simulink model "gm_parallel_min_cost_function_vopt_6phase"  (R2022a)
settings: Solver=FixedStepDiscrete  StartTime=0.0  StopTime=10.0  RelTol=1e-3
undefined symbols (not defined in the file or in its folder): f_c
libraries: hdlmdlgenlib x368
(part 1 of 3)
settings Model: Creator=Andre Merx  LastModifiedBy=Andre Merx
settings SolverCC: AlgebraicLoopSolver=TrustRegion
settings DataIOCC: LimitDataPoints=on  SaveOutput=off  SaveTime=off
settings OptimizationCC: BlockReduction=off  ConditionallyExecuteInputs=off  DefaultParameterBehavior=Inlined  LifeSpan=inf
settings DebuggingCC: AlgebraicLoopMsg=error  InheritedTsInSrcMsg=none  SingleTaskRateTransMsg=error  UnconnectedInputMsg=warning  UnconnectedOutputMsg=warning  UnconnectedLineMsg=warning  AllowSymbolicDim=off  StrictBusMsg=ErrorOnBusTreatedAsVector  SFUnexpectedBacktrackingDiag=warning  SFNoUnconditionalDefaultTransitionDiag=warning  SFExecutionAtInitializationDiag=none  SFMachineParentedDataDiag=warning  ArithmeticOperatorsInVariantConditions=warning
settings HardwareCC: ProdBitPerPointer=32  ProdBitPerSizeT=32  ProdBitPerPtrDiffT=32  ProdLargestAtomicFloat=None  ProdIntDivRoundTo=Undefined  ProdEndianess=Unspecified  ProdWordSize=32  ProdHWDeviceType=ASIC/FPGA->ASIC/FPGA  ProdEqTarget=off
settings SFSimCC: SimUseLocalCustomCode=off  CustomCodeUndefinedFunction=UseInterfaceOnly
settings RTWCC: RTWUseLocalCustomCode=off
settings CodeAppCC: StateflowObjectComments=on
settings GRTTargetCC: TargetLangStandard=C89/C90 (ANSI)
settings ConfigComp: CovScope=ReferencedModels  CovMetricSettings=dw  CovSaveCumulativeToWorkspaceVar=on  CovSaveSingleToWorkspaceVar=on  CovExternalEMLEnable=off  CovSFcnEnable=off

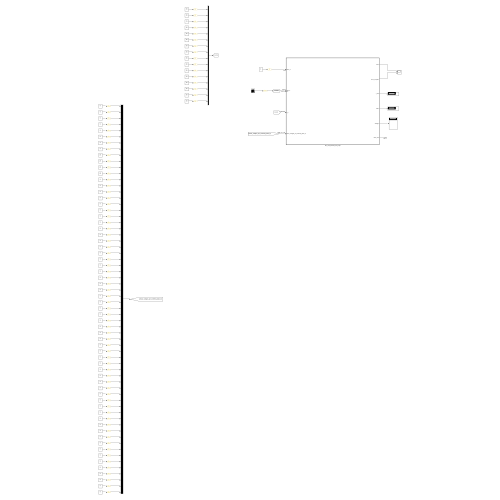
[thumbnail: Simulink's stored preview of the top-level diagram]
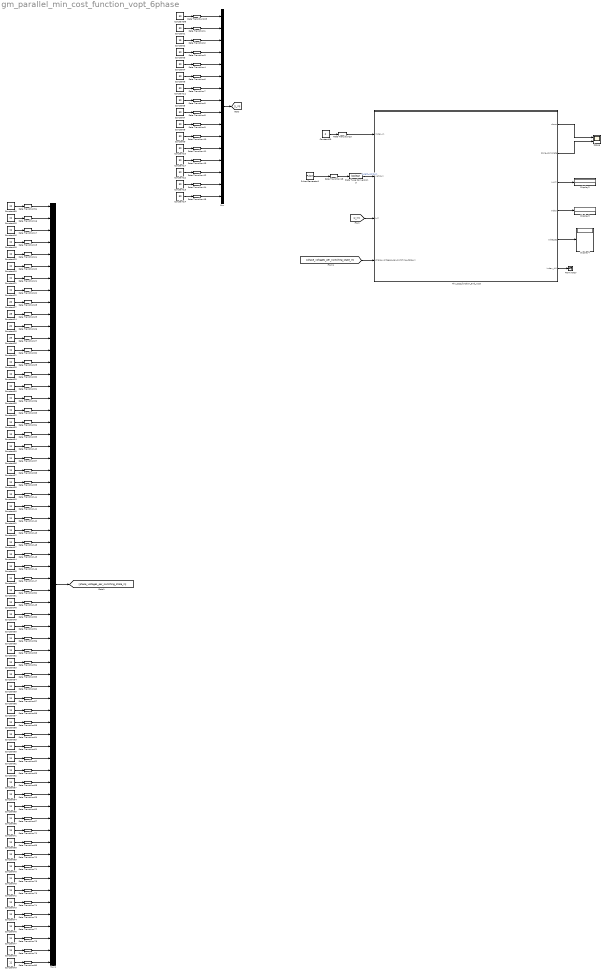
== system gm_parallel_min_cost_function_vopt_6phase ==
  Constant{1,3..14,17,98} (15 alike) : Constant  Value=30  OutDataTypeStr=fixdt(1,20,11)  SampleTime=-1
  Constant{15..16,18,20..23,28..79,89} (60 alike) : Constant  Value=11  OutDataTypeStr=fixdt(1,24,11)  SampleTime=-1  LockScale=on
  Constant19 : Constant  Value=4  OutDataTypeStr=int32  SampleTime=-1
  Constant2 : Constant  Value=15  OutDataTypeStr=fixdt(1,20,11)  SampleTime=-1
  Constant24 : Constant  Value=23  OutDataTypeStr=fixdt(1,24,11)  SampleTime=-1  LockScale=on
  Constant25 : Constant  Value=24  OutDataTypeStr=fixdt(1,24,11)  SampleTime=-1  LockScale=on
  Constant26 : Constant  Value=25  OutDataTypeStr=fixdt(1,24,11)  SampleTime=-1  LockScale=on
  Constant27 : Constant  Value=22  OutDataTypeStr=fixdt(1,24,11)  SampleTime=-1  LockScale=on
  Data Type Conversion3 : DataTypeConversion  OutDataTypeStr=boolean  SaturateOnIntegerOverflow=off  RndMeth=Floor
  Display2 : Display
  Display3 : Display
  Display4 : Display
  Min_cost_function_and_vopt : Subsystem  TreatAsAtomicUnit=on
  Mux : Mux  Inputs=16
  Mux1 : Mux  Inputs=64
  Pulse Generator1 : DiscretePulseGenerator  PulseType=Time based  Period=1/f_c
  Rate Transition{1..80,94,103} (82 alike) : RateTransition  OutPortSampleTime=Rt
  Scope : Scope  NumInputPorts=2
  Terminator : Terminator
  wires:
  Min_cost_function_and_vopt/6(Index_AXI) -> Terminator/1
  Min_cost_function_and_vopt/5(voltages) -> Display4/1
  Min_cost_function_and_vopt/4(Index) -> Display3/1
  Min_cost_function_and_vopt/3(J_AXI) -> Display2/1
  Min_cost_function_and_vopt/2(done_complete) -> Scope/2
  Min_cost_function_and_vopt/1(done) -> Scope/1
  [phase_voltages_per_switching_state_in] -> Min_cost_function_and_vopt/4(phase_voltages_per_switching_state_in)
  Mux1/1 -> [phase_voltages_per_switching_state_in]
  Rate Transition80/1 -> Mux1/64
  Rate Transition79/1 -> Mux1/63
  Rate Transition78/1 -> Mux1/62
  Rate Transition77/1 -> Mux1/61
  Rate Transition75/1 -> Mux1/60
  Rate Transition74/1 -> Mux1/59
  Rate Transition73/1 -> Mux1/58
  Rate Transition76/1 -> Mux1/57
  Rate Transition71/1 -> Mux1/56
  Rate Transition70/1 -> Mux1/55
  Rate Transition69/1 -> Mux1/54
  Rate Transition72/1 -> Mux1/53
  Rate Transition67/1 -> Mux1/52
  Rate Transition66/1 -> Mux1/51
  Rate Transition65/1 -> Mux1/50
  Rate Transition68/1 -> Mux1/49
  Rate Transition63/1 -> Mux1/48
  Rate Transition62/1 -> Mux1/47
  Rate Transition61/1 -> Mux1/46
  Rate Transition64/1 -> Mux1/45
  Rate Transition59/1 -> Mux1/44
  Rate Transition58/1 -> Mux1/43
  Rate Transition57/1 -> Mux1/42
  Rate Transition60/1 -> Mux1/41
  Rate Transition55/1 -> Mux1/40
  Rate Transition54/1 -> Mux1/39
  Rate Transition53/1 -> Mux1/38
  Rate Transition56/1 -> Mux1/37
  Rate Transition51/1 -> Mux1/36
  Rate Transition50/1 -> Mux1/35
  Rate Transition49/1 -> Mux1/34
  Rate Transition52/1 -> Mux1/33
  Rate Transition47/1 -> Mux1/32
  Rate Transition46/1 -> Mux1/31
  Rate Transition45/1 -> Mux1/30
  Rate Transition48/1 -> Mux1/29
  Rate Transition43/1 -> Mux1/28
  Rate Transition42/1 -> Mux1/27
  Rate Transition41/1 -> Mux1/26
  Rate Transition44/1 -> Mux1/25
  Rate Transition39/1 -> Mux1/24
  Rate Transition38/1 -> Mux1/23
  Rate Transition37/1 -> Mux1/22
  Rate Transition40/1 -> Mux1/21
  Rate Transition35/1 -> Mux1/20
  Rate Transition34/1 -> Mux1/19
  Rate Transition33/1 -> Mux1/18
  Rate Transition36/1 -> Mux1/17
  Rate Transition31/1 -> Mux1/16
  Rate Transition30/1 -> Mux1/15
  Rate Transition29/1 -> Mux1/14
  Rate Transition32/1 -> Mux1/13
  Rate Transition27/1 -> Mux1/12
  Rate Transition26/1 -> Mux1/11
  Rate Transition25/1 -> Mux1/10
  Rate Transition28/1 -> Mux1/9
  Rate Transition22/1 -> Mux1/8
  Rate Transition21/1 -> Mux1/7
  Rate Transition20/1 -> Mux1/6
  Rate Transition24/1 -> Mux1/5
  Rate Transition19/1 -> Mux1/4
  Rate Transition17/1 -> Mux1/3
  Rate Transition16/1 -> Mux1/2
  Rate Transition94/1 -> Mux1/1
  Constant79/1 -> Rate Transition80/1
  Constant78/1 -> Rate Transition79/1
  Constant77/1 -> Rate Transition78/1
  Constant76/1 -> Rate Transition77/1
  Constant75/1 -> Rate Transition76/1
  Constant73/1 -> Rate Transition74/1
  Constant72/1 -> Rate Transition73/1
  Constant74/1 -> Rate Transition75/1
  Constant71/1 -> Rate Transition72/1
  Constant69/1 -> Rate Transition70/1
  Constant68/1 -> Rate Transition69/1
  Constant70/1 -> Rate Transition71/1
  Constant67/1 -> Rate Transition68/1
  Constant65/1 -> Rate Transition66/1
  Constant64/1 -> Rate Transition65/1
  Constant66/1 -> Rate Transition67/1
  Constant63/1 -> Rate Transition64/1
  Constant61/1 -> Rate Transition62/1
  Constant60/1 -> Rate Transition61/1
  Constant62/1 -> Rate Transition63/1
  Constant59/1 -> Rate Transition60/1
  Constant57/1 -> Rate Transition58/1
  Constant56/1 -> Rate Transition57/1
  Constant58/1 -> Rate Transition59/1
  Constant55/1 -> Rate Transition56/1
  Constant53/1 -> Rate Transition54/1
  Constant52/1 -> Rate Transition53/1
  Constant54/1 -> Rate Transition55/1
  Constant51/1 -> Rate Transition52/1
  Constant49/1 -> Rate Transition50/1
  Constant48/1 -> Rate Transition49/1
  Constant50/1 -> Rate Transition51/1
  Constant47/1 -> Rate Transition48/1
  Constant45/1 -> Rate Transition46/1
  Constant44/1 -> Rate Transition45/1
  Constant46/1 -> Rate Transition47/1
  Constant43/1 -> Rate Transition44/1
  Constant41/1 -> Rate Transition42/1
  Constant40/1 -> Rate Transition41/1
  Constant42/1 -> Rate Transition43/1
  Constant39/1 -> Rate Transition40/1
  Constant37/1 -> Rate Transition38/1
  Constant36/1 -> Rate Transition37/1
  Constant38/1 -> Rate Transition39/1
  Constant35/1 -> Rate Transition36/1
  Constant33/1 -> Rate Transition34/1
  Constant32/1 -> Rate Transition33/1
  Constant34/1 -> Rate Transition35/1
  Constant31/1 -> Rate Transition32/1
  Constant29/1 -> Rate Transition30/1
  Constant28/1 -> Rate Transition29/1
  Constant30/1 -> Rate Transition31/1
  Constant27/1 -> Rate Transition28/1
  Constant25/1 -> Rate Transition26/1
  Constant24/1 -> Rate Transition25/1
  Constant26/1 -> Rate Transition27/1
  Constant23/1 -> Rate Transition24/1
  Constant21/1 -> Rate Transition21/1
  Constant20/1 -> Rate Transition20/1
  Constant22/1 -> Rate Transition22/1
  Constant18/1 -> Rate Transition19/1
  Constant16/1 -> Rate Transition17/1
  Constant15/1 -> Rate Transition16/1
  Constant89/1 -> Rate Transition94/1
  [J_in] -> Min_cost_function_and_vopt/3(J_in)
  Mux/1 -> [J_in]
  Rate Transition12/1 -> Mux/14
  Constant17/1 -> Rate Transition13/1
  Constant12/1 -> Rate Transition12/1
  Rate Transition13/1 -> Mux/13
  Rate Transition15/1 -> Mux/16
  Constant14/1 -> Rate Transition15/1
  Constant13/1 -> Rate Transition14/1
  Rate Transition14/1 -> Mux/15
  Rate Transition5/1 -> Mux/8
  Constant11/1 -> Rate Transition7/1
  Constant5/1 -> Rate Transition5/1
  Rate Transition7/1 -> Mux/7
  Rate Transition11/1 -> Mux/12
  Rate Transition9/1 -> Mux/10
  Constant8/1 -> Rate Transition9/1
  Constant10/1 -> Rate Transition11/1
  Rate Transition10/1 -> Mux/11
  Constant9/1 -> Rate Transition10/1
  Constant7/1 -> Rate Transition8/1
  Rate Transition8/1 -> Mux/9
  Rate Transition6/1 -> Mux/6
  Constant6/1 -> Rate Transition6/1
  Rate Transition4/1 -> Mux/5
  Constant4/1 -> Rate Transition4/1
  Rate Transition3/1 -> Mux/4
  Constant3/1 -> Rate Transition3/1
  Rate Transition2/1 -> Mux/3
  Constant2/1 -> Rate Transition2/1
  Rate Transition1/1 -> Mux/2
  Constant1/1 -> Rate Transition1/1
  Rate Transition103/1 -> Mux/1
  Constant98/1 -> Rate Transition103/1
  Pulse Generator1/1 -> Rate Transition18/1
  Data Type Conversion3/1 -> Min_cost_function_and_vopt/2(valid_in)  "curent_valid_in"
  Rate Transition18/1 -> Data Type Conversion3/1
  Constant19/1 -> Rate Transition23/1
  Rate Transition23/1 -> Min_cost_function_and_vopt/1(Index_in)
